simulink model "simscape_robot_delta_v8"  (R2024b)
settings: Solver=ode15s  StartTime=0.0  StopTime=20.0  FixedStep=1e-3  RelTol=1e-3
model workspace (MAT data in the model file):
  kd1 = 14
  kd2 = 13.6
  kd3 = 37.9
  ki1 = 39
  ki2 = 36
  ki3 = 11.6
  kp1 = 12.6
  kp2 = 12.2
  kp3 = 14.4
values from neighbouring files (symbols this model uses):
  N = floor(size(err,1)/window)    [grafica_error.m]
undefined symbols (not defined in the file or in its folder): X, Y, Z
libraries: sm_lib x72, nesl_utility x7
(part 1 of 3)
settings Model: Creator=rodri  LastModifiedBy=rodri

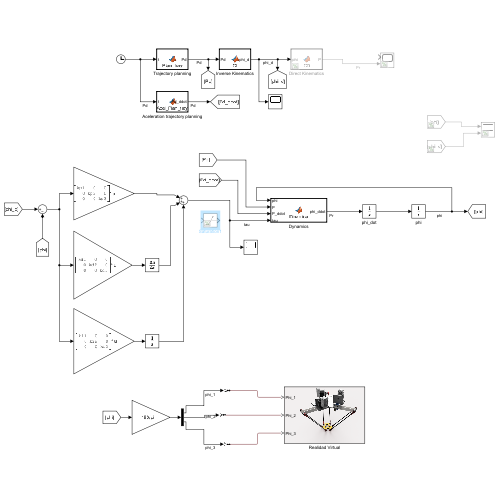
[thumbnail: Simulink's stored preview of the top-level diagram]
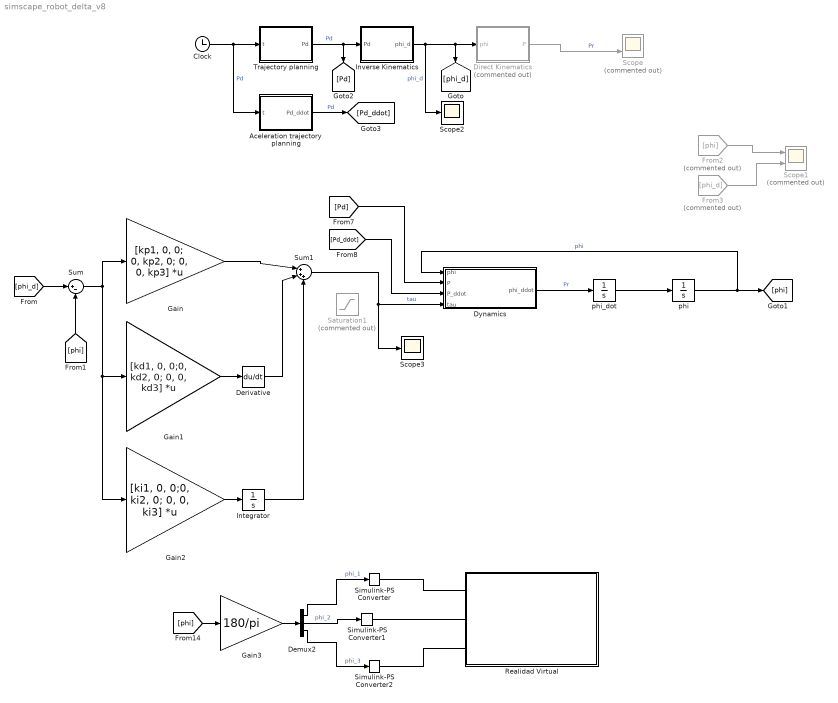
== system simscape_robot_delta_v8 ==
  Aceleration trajectory planning : MATLAB Function  TreatAsAtomicUnit=on
  Clock : Clock
  Demux2 : Demux  Outputs=3
  Derivative : Derivative
  Direct Kinematics : MATLAB Function  Commented=on  TreatAsAtomicUnit=on
  Dynamics : MATLAB Function  TreatAsAtomicUnit=on
  From2 : From  Commented=on  GotoTag=phi
  From3 : From  Commented=on  GotoTag=phi_d
  Gain : Gain  Gain=[kp1, 0, 0; 0, kp2, 0; 0, 0, kp3]  Multiplication=Matrix(K*u)
  Gain1 : Gain  Gain=[kd1, 0, 0;0, kd2, 0; 0, 0, kd3]  Multiplication=Matrix(K*u)
  Gain2 : Gain  Gain=[ki1, 0, 0;0, ki2, 0; 0, 0, ki3]  Multiplication=Matrix(K*u)
  Gain3 : Gain  Gain=180/pi
  Integrator : Integrator  InitialCondition=[0;0;0]
  Inverse Kinematics : MATLAB Function  TreatAsAtomicUnit=on
  Realidad Virtual : Subsystem
      mask Display: image('robot_delta_azucena.png');
  Saturation1 : Saturate  Commented=on  UpperLimit=19.8  LowerLimit=-19.8
  Scope : Scope  Commented=on  NumInputPorts=2
  Scope1 : Scope  Commented=on  NumInputPorts=2
  Scope2 : Scope
  Scope3 : Scope
  Simulink-PS Converter : nesl_utility/Simulink-PS Converter  PhysicalDomain=network_engine_domain  SubClassName=ps_input  LeftPortType=input  RightPortType=output  PseudoPeriodic=off  Frequencies=[]  NoiseDistribution=none  NoiseParameters=[]  Unit=deg  AffineConversion=off  FilteringAndDerivatives=filter  SimscapeFilterOrder=2  InputFilterTimeConstant=0.001  UdotUserProvided=0
  Simulink-PS Converter1 : nesl_utility/Simulink-PS Converter  PhysicalDomain=network_engine_domain  SubClassName=ps_input  LeftPortType=input  RightPortType=output  PseudoPeriodic=off  Frequencies=[]  NoiseDistribution=none  NoiseParameters=[]  Unit=deg  AffineConversion=off  FilteringAndDerivatives=filter  SimscapeFilterOrder=2  InputFilterTimeConstant=0.001  UdotUserProvided=0
  Simulink-PS Converter2 : nesl_utility/Simulink-PS Converter  PhysicalDomain=network_engine_domain  SubClassName=ps_input  LeftPortType=input  RightPortType=output  PseudoPeriodic=off  Frequencies=[]  NoiseDistribution=none  NoiseParameters=[]  Unit=deg  AffineConversion=off  FilteringAndDerivatives=filter  SimscapeFilterOrder=2  InputFilterTimeConstant=0.001  UdotUserProvided=0
  Sum : Sum  Inputs=|+-
  Sum1 : Sum  Inputs=|+++
  Trajectory planning : MATLAB Function  TreatAsAtomicUnit=on
  phi : Integrator  InitialCondition=[0;0;0]
  phi_dot : Integrator  InitialCondition=[0;0;0]
  wires:
  Sum/1 -> Gain2/1, Gain1/1, Gain/1
  Gain/1 -> Sum1/1
  Derivative/1 -> Sum1/2
  [Pd] -> Dynamics/2(P)
  Clock/1 -> Aceleration trajectory planning/1(t), Trajectory planning/1(t)  "Pd"
  phi/1 -> Dynamics/1(phi), [phi]  "phi"
  Direct Kinematics/1(P) -> Scope/2  "Pr"
  Integrator/1 -> Sum1/3
  [Pd_ddot] -> Dynamics/3(P_ddot)
  Sum1/1 -> Scope3/1, Dynamics/4(tau)  "tau"
  Gain1/1 -> Derivative/1
  [phi_d] -> Sum/1
  Trajectory planning/1(Pd) -> Inverse Kinematics/1(Pd), [Pd]  "Pd"
  From3/1 -> Scope1/2
  Dynamics/1(phi_ddot) -> phi_dot/1  "Pr"
  Gain2/1 -> Integrator/1
  phi_dot/1 -> phi/1
  Inverse Kinematics/1(phi_d) -> Scope2/1, [phi_d], Direct Kinematics/1(phi)  "phi_d"
  Aceleration trajectory planning/1(Pd_ddot) -> [Pd_ddot]  "Pd"
  From2/1 -> Scope1/1
  [phi] -> Sum/2
  Demux2/1 -> Simulink-PS Converter/1  "phi_1"
  [phi] -> Gain3/1
  Gain3/1 -> Demux2/1
  Demux2/3 -> Simulink-PS Converter2/1  "phi_3"
  Demux2/2 -> Simulink-PS Converter1/1  "phi_2"
  connections:
  Simulink-PS Converter/RConn1 -- Realidad Virtual/LConn1
  Simulink-PS Converter1/RConn1 -- Realidad Virtual/LConn2
  Simulink-PS Converter2/RConn1 -- Realidad Virtual/LConn3
